simulink model "resonant_dc_link"  (Simulink 6.1)
settings: Solver=ode23tb  StartTime=0.0  StopTime=1e-3  MaxStep=1e-7  RelTol=1e-4  AbsTol=1e-4
libraries: powerlib x6
settings Model: Creator=dkennedy  LastModifiedBy=ThinkPad  ExtModeTrigMode=oneshot  ExtModeArmWhenConnect=off  ExtModeAutoUpdateStatusClock=off
settings DataIOCC: LimitDataPoints=off  SignalLoggingName=sigsOut
settings OptimizationCC: BlockReduction=off  BooleanDataType=off
settings HardwareCC: TargetUnknown=on

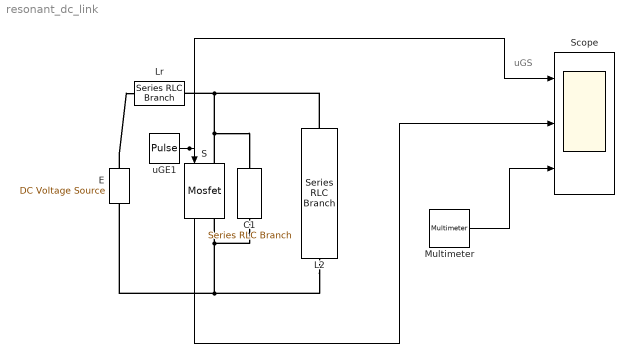
== system resonant_dc_link ==
  note: uGS
  C1 : powerlib/Elements/Series RLC Branch  Orientation=down  PhysicalDomain=powersysdomain  SubClassName=unknown  LeftPortType=p1  RightPortType=p1  LConnTagsString=__new0  RConnTagsString=__new0  Resistance=0  Inductance=0  Capacitance=1e-6  Measurements=Branch voltage
  E : powerlib/Electrical Sources/DC Voltage Source  Description=source block  Orientation=up  Amplitude=50  Measurements=None
      settings: AttributesFormatString=\n
  L2 : powerlib/Elements/Series RLC Branch  Orientation=down  PhysicalDomain=powersysdomain  SubClassName=unknown  LeftPortType=p1  RightPortType=p1  LConnTagsString=__new0  RConnTagsString=__new0  Resistance=1  Inductance=1e-3  Capacitance=inf  Measurements=Branch current
  Lr : powerlib/Elements/Series RLC Branch  PhysicalDomain=powersysdomain  SubClassName=unknown  LeftPortType=p1  RightPortType=p1  LConnTagsString=__new0  RConnTagsString=__new0  Resistance=0  Inductance=1e-5  Capacitance=inf  Measurements=Branch current
  Multimeter : powerlib/Measurements/Multimeter  PhasorSimulation=off  OutputType=Complex  sel=[2 3]  L=3  Gain=[1 1]  yselected={'Ib: L2','Ib: Lr'};  PSBOutputType=1  PSBequivalent=0  AxesSetting=[0,0.1,-100,100]  Display=0  SavedBlockNames=-11
  S : powerlib/Power Electronics/Mosfet  Orientation=down  Ron=0.01  Lon=1e-9  Rd=.1  IC=0  Rs=100  Cs=0  Measurements=on
  Scope : Scope  NumInputPorts=3
      settings: TimeRange=0.0001  YMin=-0.5~-50~0  YMax=1.5~150~100  SaveName=var  MaxDataPoints=50000
  uGE1 : DiscretePulseGenerator  PulseType=Time based  Period=20e-6  PulseWidth=10
  wires:
  uGE1/1 -> S/1, Scope/1
  S/1 -> Scope/2
  Multimeter/1 -> Scope/3
  connections:
  L2/RConn1 -- S/RConn1 -- C1/RConn1 -- E/LConn1
  E/RConn1 -- Lr/LConn1
  S/LConn1 -- C1/LConn1 -- Lr/RConn1 -- L2/LConn1
